simulink library "FixedAttenuatorLib"  (R2022b)
settings: Solver=VariableStepAuto  StartTime=0.0  StopTime=10.0  RelTol=1e-3
undefined symbols (not defined in the file): Row
libraries: TuneVar x2, TOP x1, HandyTextFile x1
settings Model: Creator=sa1045272  LastModifiedBy=sa1045272
settings SolverCC: AlgebraicLoopSolver=TrustRegion
settings DebuggingCC: UnconnectedInputMsg=warning  UnconnectedOutputMsg=warning  UnconnectedLineMsg=warning  SFMachineParentedDataDiag=warning
settings ModelReferenceCC: EnableRefExpFcnMdlSchedulingChecks=on

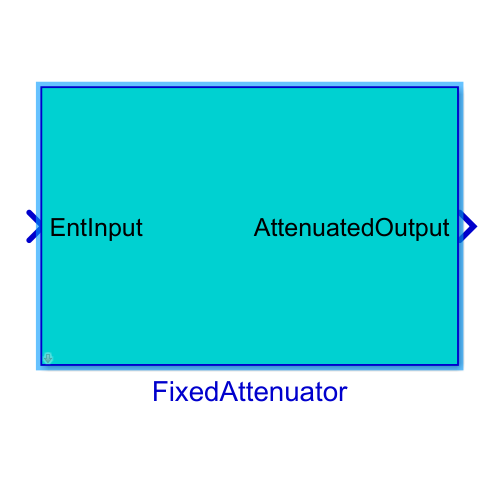
[thumbnail: Simulink's stored preview of the top-level diagram]
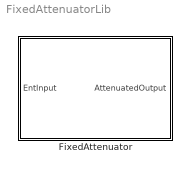
== system FixedAttenuatorLib ==
  FixedAttenuator : Subsystem  mask{Config=[]}
      mask prompts: Config "FixedAttenuatorConfig"
      mask init:
      | blkh=gcbh;
      | Config=BTConfig.Assert(blkh,Config);
      | 
      | Config.Validate();
      | Config.DoMaskInit(blkh);
      mask DialogControl ClassContainer Prompt: Fixed Attenuator Class Instance

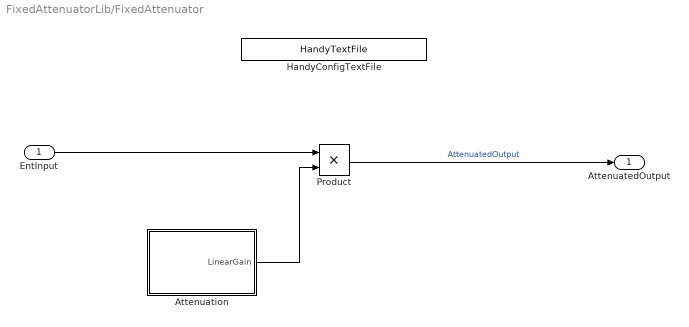
== system FixedAttenuatorLib/FixedAttenuator ==
  EntInput : Inport
  "Attenuation " : Subsystem
  HandyConfigTextFile : HandyTextFile/HandyTextFile  TemplateSource=Config  FileSuffix=File  OpenDialogOnLoad=off  UseThisBlockName=off  AddGrandParentNamePrefix=off  TheDefaultText=% $(FILENAME) $(PREFIX) $(SUFFIX)  ShowInLibBrowser=on
      settings: SourceProductName=Bose Talaria
  Product : Product
  AttenuatedOutput : Outport
  wires:
  Product/1 -> AttenuatedOutput/1  "AttenuatedOutput"
  "Attenuation "/1(LinearGain) -> Product/2
  EntInput/1 -> Product/1

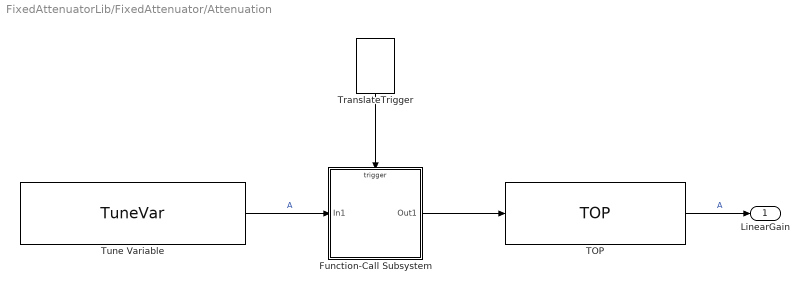
== system FixedAttenuatorLib/FixedAttenuator/Attenuation  ==
  Function-Call Subsystem : Subsystem  TreatAsAtomicUnit=on
  TOP : TOP/TOP  TriggerInit=[380 164 560 226]  TopName=A  DataType=single  BankNumber=0  PreOverlay=false  PostOverlay=false  Role=Automatic
      settings: SourceProductName=Bose Talaria
  TranslateTrigger : TuneVar/TranslateTrigger  TriggerInit=[-809 110 -771 165]
      settings: SourceProductName=Bose Talaria
  Tune Variable : TuneVar/TuneVar  TuneName=A  SpecifyMaxSize=off  VariableDim=1 (Row)  MaxSize=[1 1]  TunabilityNumber=1  MinValue=[]  MaxValue=[]  TriggerInit=[-105 164 120 226]  MaskValue=Config.A
      settings: SourceProductName=Bose Talaria
  LinearGain : Outport
  wires:
  Function-Call Subsystem/1(Out1) -> TOP/1
  Tune Variable/1 -> Function-Call Subsystem/1(In1)  "A"
  TranslateTrigger/1 -> Function-Call Subsystem/Trigger
  TOP/1 -> LinearGain/1  "A"

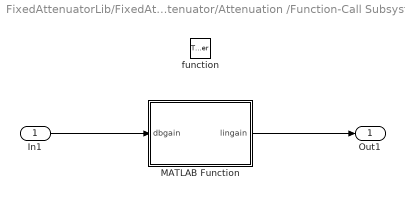
== system FixedAttenuatorLib/FixedAttenuator/Attenuation /Function-Call Subsystem ==
  In1 : Inport
  function : TriggerPort  TriggerType=function-call  VariantControl=Variant
  MATLAB Function : MATLAB Function  TreatAsAtomicUnit=on
  Out1 : Outport
  wires:
  In1/1 -> MATLAB Function/1(dbgain)
  MATLAB Function/1(lingain) -> Out1/1

== matlab function FixedAttenuatorLib/FixedAttenuator/Attenuation /Function-Call Subsystem/MATLAB Function ==
  data: dbgain input; lingain output
function lingain = fcn(dbgain)
    lingain = 10^(dbgain.Value/20);   
end
